simulink model "K_identification"  (R2021a)
settings: Solver=VariableStepAuto  StartTime=0.0  StopTime=170  RelTol=1e-3
settings Model: Creator=matij  LastModifiedBy=matij

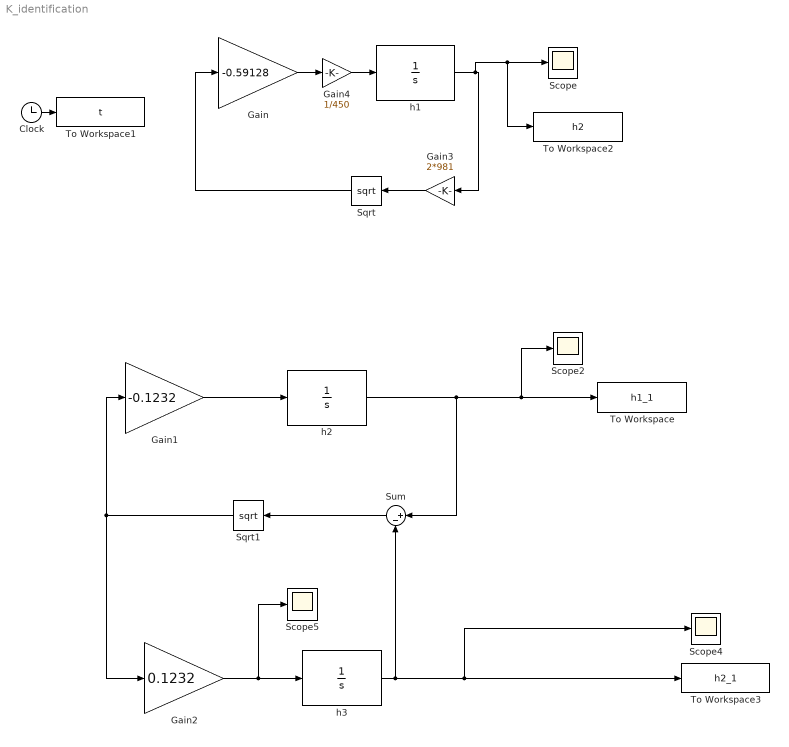
== system K_identification ==
  Clock : Clock
  Gain : Gain  Gain=-0.59128
  Gain1 : Gain  Gain=-0.1232
  Gain2 : Gain  Gain=0.1232
  Gain3 : Gain  Gain=2*981
  Gain4 : Gain  Gain=1/450
  Scope{,2,4..5} (4 alike) : Scope
  Sqrt : Sqrt  SaturateOnIntegerOverflow=on
  Sqrt1 : Sqrt  SaturateOnIntegerOverflow=on
  Sum : Sum  Inputs=|+-
  To Workspace : ToWorkspace  VariableName=h1_1  SampleTime=0.01
  To Workspace1 : ToWorkspace  VariableName=t  SampleTime=0.01
  To Workspace2 : ToWorkspace  VariableName=h2  SampleTime=0.01
  To Workspace3 : ToWorkspace  VariableName=h2_1  SampleTime=0.01
  h1 : Integrator  InitialCondition=25
  h2 : Integrator  InitialCondition=32
  h3 : Integrator  InitialCondition=5
  wires:
  Clock/1 -> To Workspace1/1
  Sqrt/1 -> Gain/1
  Gain/1 -> Gain4/1
  h1/1 -> To Workspace2/1, Scope/1, Gain3/1
  Gain1/1 -> h2/1
  Gain2/1 -> Scope5/1, h3/1
  h3/1 -> Scope4/1, To Workspace3/1, Sum/2
  Sqrt1/1 -> Gain2/1, Gain1/1
  h2/1 -> Scope2/1, To Workspace/1, Sum/1
  Sum/1 -> Sqrt1/1
  Gain3/1 -> Sqrt/1
  Gain4/1 -> h1/1
